simulink model "BangBang"  (R2022b)
settings: Solver=FixedStepDiscrete  StartTime=0.0  StopTime=1  FixedStep=0.000001  RelTol=1e-3
settings Model: Creator=yll  LastModifiedBy=yll

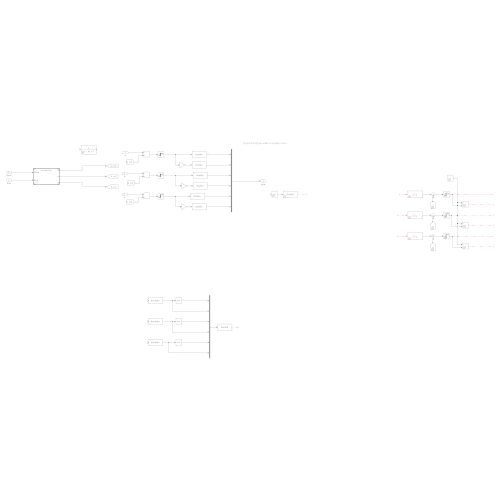
[thumbnail: Simulink's stored preview of the top-level diagram]
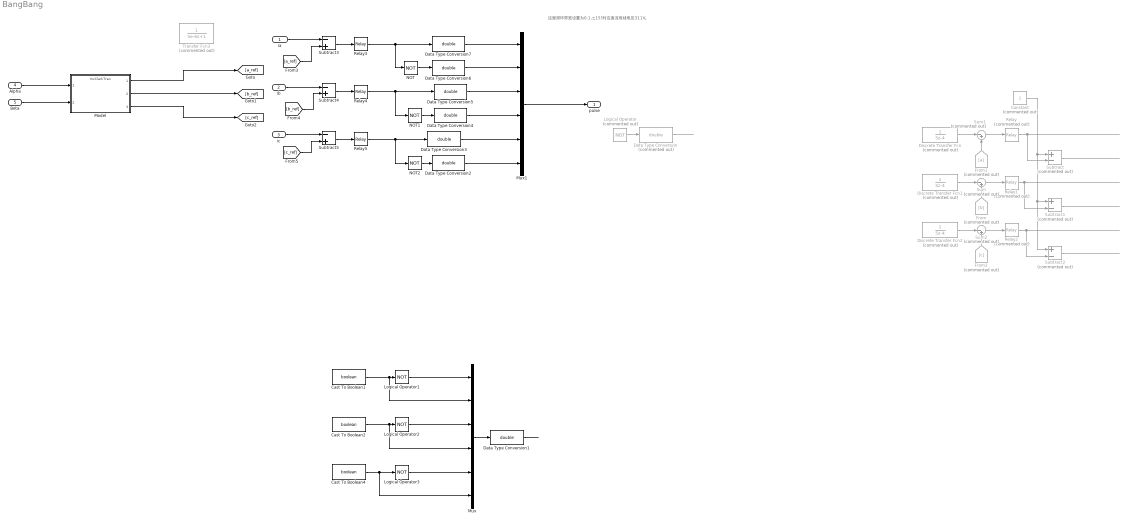
== system BangBang ==
  note: 这里滞环带宽设置为0.1,±155对应直流母线电压311V。
  ia : Inport
  ib : Inport  Port=2
  ic : Inport  Port=3
  Alpha : Inport  Port=4
  Beta : Inport  Port=5
  Cast To Boolean1 : DataTypeConversion  OutDataTypeStr=boolean  SaturateOnIntegerOverflow=off  RndMeth=Floor
  Cast To Boolean2 : DataTypeConversion  OutDataTypeStr=boolean  SaturateOnIntegerOverflow=off  RndMeth=Floor
  Cast To Boolean4 : DataTypeConversion  OutDataTypeStr=boolean  SaturateOnIntegerOverflow=off  RndMeth=Floor
  Constant : Constant  Commented=on
  Data Type Conversion : DataTypeConversion  Commented=on  OutDataTypeStr=double  SaturateOnIntegerOverflow=off  RndMeth=Floor
  Data Type Conversion{1..7} (7 alike) : DataTypeConversion  OutDataTypeStr=double  SaturateOnIntegerOverflow=off  RndMeth=Floor
  Discrete Transfer Fcn : DiscreteTransferFcn  Commented=on  Denominator=[5 -4]
  Discrete Transfer Fcn1 : DiscreteTransferFcn  Commented=on  Denominator=[5 -4]
  Discrete Transfer Fcn2 : DiscreteTransferFcn  Commented=on  Denominator=[5 -4]
  From : From  Commented=on  GotoTag=b
  From1 : From  Commented=on  GotoTag=a
  From2 : From  Commented=on  GotoTag=c
  Logical Operator : Logic  Commented=on  Operator=NOT  AllPortsSameDT=off  OutDataTypeStr=boolean
  Logical Operator1 : Logic  Operator=NOT  AllPortsSameDT=off  OutDataTypeStr=boolean
  Logical Operator2 : Logic  Operator=NOT  AllPortsSameDT=off  OutDataTypeStr=boolean
  Logical Operator3 : Logic  Operator=NOT  AllPortsSameDT=off  OutDataTypeStr=boolean
  Model : ModelReference  ModelNameDialog=InvClarkTran.slx  SimulationMode=Normal  ModelReferenceVersion=1.6
  Mux : Mux  Inputs=6
  Mux1 : Mux  Inputs=6
  NOT : Logic  Operator=NOT  IconShape=distinctive  AllPortsSameDT=off  OutDataTypeStr=boolean
  NOT1 : Logic  Operator=NOT  IconShape=distinctive  AllPortsSameDT=off  OutDataTypeStr=boolean
  NOT2 : Logic  Operator=NOT  IconShape=distinctive  AllPortsSameDT=off  OutDataTypeStr=boolean
  Relay : Relay  Commented=on  OnSwitchValue=0.05  OffSwitchValue=-0.05  OnOutputValue=155  OffOutputValue=-155
  Relay1 : Relay  Commented=on  OnSwitchValue=0.05  OffSwitchValue=-0.05  OnOutputValue=155  OffOutputValue=-155
  Relay2 : Relay  Commented=on  OnSwitchValue=0.05  OffSwitchValue=-0.05  OnOutputValue=155  OffOutputValue=-155
  Relay3 : Relay  OnSwitchValue=0.001  OffSwitchValue=-0.001
  Relay4 : Relay  OnSwitchValue=0.001  OffSwitchValue=-0.001
  Relay5 : Relay  OnSwitchValue=0.001  OffSwitchValue=-0.001
  Subtract : Sum  Commented=on  Inputs=+-
  Subtract1 : Sum  Commented=on  Inputs=+-
  Subtract2 : Sum  Commented=on  Inputs=+-
  Subtract3 : Sum  Inputs=-+
  Subtract4 : Sum  Inputs=-+
  Subtract5 : Sum  Inputs=-+
  Sum : Sum  Commented=on  Inputs=|-+
  Sum1 : Sum  Commented=on  Inputs=|-+
  Sum2 : Sum  Commented=on  Inputs=|-+
  Transfer Fcn3 : TransferFcn  Commented=on  Denominator=[5e-6 1]
  pulse : Outport
  wires:
  Alpha/1 -> Model/1
  Beta/1 -> Model/2
  Logical Operator/1 -> Data Type Conversion/1
  Data Type Conversion/1 -> ?
  Relay2/1 -> Subtract2/2
  Sum2/1 -> Relay2/1
  Subtract1/1 -> ?
  Subtract/1 -> ?
  Discrete Transfer Fcn/1 -> Sum1/1
  ? -> Discrete Transfer Fcn2/1
  Discrete Transfer Fcn2/1 -> Sum2/1
  ? -> Discrete Transfer Fcn1/1
  Sum/1 -> Relay1/1
  Relay1/1 -> Subtract1/2
  From1/1 -> Sum1/2
  ? -> Discrete Transfer Fcn/1
  From/1 -> Sum/2
  Subtract2/1 -> ?
  From2/1 -> Sum2/2
  Discrete Transfer Fcn1/1 -> Sum/1
  Sum1/1 -> Relay/1
  Constant/1 -> Subtract1/1, Subtract2/1, Subtract/1
  Relay/1 -> Subtract/2
  [a_ref] -> Subtract3/2
  [b_ref] -> Subtract4/2
  [c_ref] -> Subtract5/2
  Subtract3/1 -> Relay3/1
  Subtract4/1 -> Relay4/1
  Subtract5/1 -> Relay5/1
  ia/1 -> Subtract3/1
  ib/1 -> Subtract4/1
  ic/1 -> Subtract5/1
  Cast To Boolean1/1 -> Mux/2, Logical Operator1/1
  Logical Operator1/1 -> Mux/1
  Mux/1 -> Data Type Conversion1/1
  Logical Operator3/1 -> Mux/5
  Cast To Boolean4/1 -> Mux/6, Logical Operator3/1
  Cast To Boolean2/1 -> Mux/4, Logical Operator2/1
  Data Type Conversion1/1 -> ?
  Logical Operator2/1 -> Mux/3
  Relay5/1 -> NOT2/1, Data Type Conversion3/1
  Mux1/1 -> pulse/1
  Relay3/1 -> NOT/1, Data Type Conversion7/1
  Relay4/1 -> NOT1/1, Data Type Conversion5/1
  NOT/1 -> Data Type Conversion6/1
  NOT1/1 -> Data Type Conversion4/1
  NOT2/1 -> Data Type Conversion2/1
  Data Type Conversion2/1 -> Mux1/6
  Data Type Conversion3/1 -> Mux1/5
  Data Type Conversion4/1 -> Mux1/4
  Data Type Conversion5/1 -> Mux1/3
  Data Type Conversion6/1 -> Mux1/2
  Data Type Conversion7/1 -> Mux1/1
  Model/1 -> [a_ref]
  Model/2 -> [b_ref]
  Model/3 -> [c_ref]
